simulink model "test_turb_sub"  (R2016a)
settings: Solver=VariableStepAuto  StartTime=0.0  StopTime=20  MaxStep=1e-3  RelTol=1e-3
libraries: simCryogenics_lib x12, nesl_utility x12, simulink x1
settings Model: Creator=FB229602  LastModifiedBy=FB229602
settings SimscapeCC: SimscapeLogType=all  SimscapeLogLimitData=off

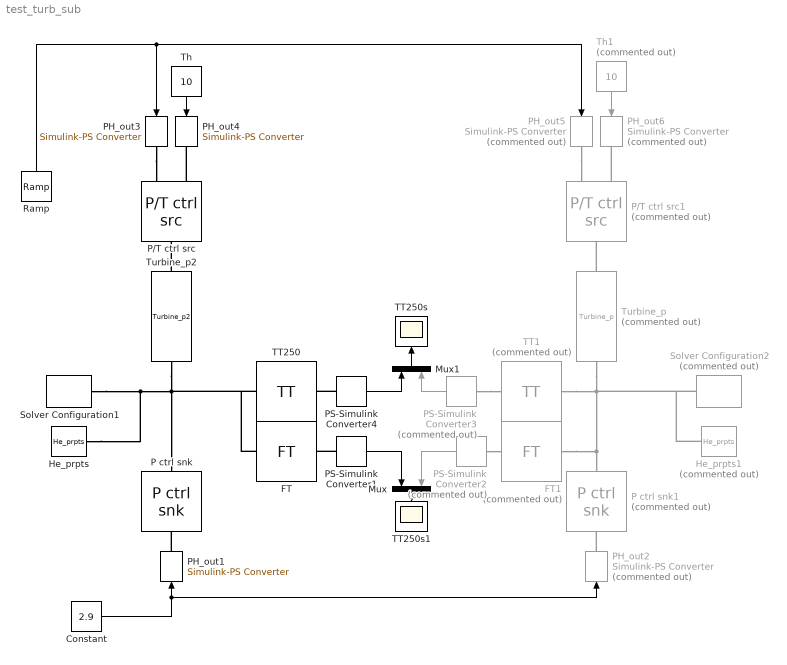
== system test_turb_sub ==
  Constant : Constant  Value=2.9
  FT : simCryogenics_lib/Sensors/FT
  FT1 : simCryogenics_lib/Sensors/FT  Commented=on
  He_prpts : simCryogenics_lib/Utilities/He_prpts  P_min=0.25 bar  P_max=20 bar  T_min=3 K  T_max=320 K  N=100  Mol=4.0026 * 10 ^ (- 3) kg/mol
  He_prpts1 : simCryogenics_lib/Utilities/He_prpts  Commented=on  P_min=0.25 bar  P_max=20 bar  T_min=3 K  T_max=320 K  N=100  Mol=4.0026 * 10 ^ (- 3) kg/mol
  Mux : Mux  Inputs=2
  Mux1 : Mux  Inputs=2
  P ctrl snk : simCryogenics_lib/Sources_Sinks/P ctrl snk
  P ctrl snk1 : simCryogenics_lib/Sources_Sinks/P ctrl snk  Commented=on
  P/T ctrl src : simCryogenics_lib/Sources_Sinks/P//T ctrl src
  P/T ctrl src1 : simCryogenics_lib/Sources_Sinks/P//T ctrl src  Commented=on
  PH_out1 : nesl_utility/Simulink-PS Converter  PhysicalDomain=network_engine_domain  SubClassName=ps_input  LeftPortType=input  RightPortType=output  PseudoPeriodic=off  Frequencies=[]  NoiseDistribution=none  NoiseParameters=[]  Unit=1  AffineConversion=off  InputFiltering=off  SimscapeFilterOrder=1  InputFilterTimeConstant=0.001  UdotUserProvided=1
  PH_out2 : nesl_utility/Simulink-PS Converter  Commented=on  PhysicalDomain=network_engine_domain  SubClassName=ps_input  LeftPortType=input  RightPortType=output  PseudoPeriodic=off  Frequencies=[]  NoiseDistribution=none  NoiseParameters=[]  Unit=1  AffineConversion=off  InputFiltering=off  SimscapeFilterOrder=1  InputFilterTimeConstant=0.001  UdotUserProvided=1
  PH_out3 : nesl_utility/Simulink-PS Converter  PhysicalDomain=network_engine_domain  SubClassName=ps_input  LeftPortType=input  RightPortType=output  PseudoPeriodic=off  Frequencies=[]  NoiseDistribution=none  NoiseParameters=[]  Unit=bar  AffineConversion=off  InputFiltering=off  SimscapeFilterOrder=1  InputFilterTimeConstant=0.001  UdotUserProvided=1
  PH_out4 : nesl_utility/Simulink-PS Converter  PhysicalDomain=network_engine_domain  SubClassName=ps_input  LeftPortType=input  RightPortType=output  PseudoPeriodic=off  Frequencies=[]  NoiseDistribution=none  NoiseParameters=[]  Unit=K  AffineConversion=off  InputFiltering=off  SimscapeFilterOrder=1  InputFilterTimeConstant=0.001  UdotUserProvided=1
  PH_out5 : nesl_utility/Simulink-PS Converter  Commented=on  PhysicalDomain=network_engine_domain  SubClassName=ps_input  LeftPortType=input  RightPortType=output  PseudoPeriodic=off  Frequencies=[]  NoiseDistribution=none  NoiseParameters=[]  Unit=bar  AffineConversion=off  InputFiltering=off  SimscapeFilterOrder=1  InputFilterTimeConstant=0.001  UdotUserProvided=1
  PH_out6 : nesl_utility/Simulink-PS Converter  Commented=on  PhysicalDomain=network_engine_domain  SubClassName=ps_input  LeftPortType=input  RightPortType=output  PseudoPeriodic=off  Frequencies=[]  NoiseDistribution=none  NoiseParameters=[]  Unit=K  AffineConversion=off  InputFiltering=off  SimscapeFilterOrder=1  InputFilterTimeConstant=0.001  UdotUserProvided=1
  PS-Simulink Converter1 : nesl_utility/PS-Simulink Converter  PhysicalDomain=network_engine_domain  SubClassName=ps_output  LeftPortType=input  RightPortType=output  PseudoPeriodic=off  Frequencies=[]  Unit=1  AffineConversion=off
  PS-Simulink Converter2 : nesl_utility/PS-Simulink Converter  Commented=on  PhysicalDomain=network_engine_domain  SubClassName=ps_output  LeftPortType=input  RightPortType=output  PseudoPeriodic=off  Frequencies=[]  Unit=1  AffineConversion=off
  PS-Simulink Converter3 : nesl_utility/PS-Simulink Converter  Commented=on  PhysicalDomain=network_engine_domain  SubClassName=ps_output  LeftPortType=input  RightPortType=output  PseudoPeriodic=off  Frequencies=[]  Unit=1  AffineConversion=off
  PS-Simulink Converter4 : nesl_utility/PS-Simulink Converter  PhysicalDomain=network_engine_domain  SubClassName=ps_output  LeftPortType=input  RightPortType=output  PseudoPeriodic=off  Frequencies=[]  Unit=1  AffineConversion=off
  Ramp : simulink/Sources/Ramp  slope=-1  start=0  X0=18
  Solver Configuration1 : nesl_utility/Solver Configuration  PhysicalDomain=network_engine_domain  SubClassName=solver  LeftPortType=input  RightPortType=generic  Accelerate=off  Tones=[]  Harmonics=[]  SimulateNoise=off  Profile=off  UseLocalSampling=off  EnableSwitchedLinearOptims=on  FrequencyDomain=off  UseCCode=off  RelTol=0.001  AbsTol=1e-06  MinStep=1e-09  ToWorkspace=off  RevertToSquareIcSolve=off  NumHomotopyIterations=100  PhasorMode=off  PhasorModeNumHarmonics=1  OverrideAbsTol=off  DoDC=off  ResidualTolerance=1e-09  UseLocalSolver=off  LocalSolverChoice=NE_BACKWARD_EULER_ADVANCER  LocalSolverSampleTime=20  DoFixedCost=off  MaxNonlinIter=10  MaxModeIter=2  LinearAlgebra=Sparse  DelaysMemoryBudget=1024  AutomaticFiltering=on  FilteringTimeConstant=0.001
  Solver Configuration2 : nesl_utility/Solver Configuration  Commented=on  PhysicalDomain=network_engine_domain  SubClassName=solver  LeftPortType=input  RightPortType=generic  Accelerate=off  Tones=[]  Harmonics=[]  SimulateNoise=off  Profile=off  UseLocalSampling=off  EnableSwitchedLinearOptims=on  FrequencyDomain=off  UseCCode=off  RelTol=0.001  AbsTol=1e-06  MinStep=1e-09  ToWorkspace=off  RevertToSquareIcSolve=off  NumHomotopyIterations=100  PhasorMode=off  PhasorModeNumHarmonics=1  OverrideAbsTol=off  DoDC=off  ResidualTolerance=1e-09  UseLocalSolver=off  LocalSolverChoice=NE_BACKWARD_EULER_ADVANCER  LocalSolverSampleTime=20  DoFixedCost=off  MaxNonlinIter=10  MaxModeIter=2  LinearAlgebra=Sparse  DelaysMemoryBudget=1024  AutomaticFiltering=on  FilteringTimeConstant=0.001
  TT1 : simCryogenics_lib/Sensors/TT  Commented=on
  TT250 : simCryogenics_lib/Sensors/TT
  TT250s : Scope
  TT250s1 : Scope
  Th : Constant  Value=10
  Th1 : Constant  Commented=on  Value=10
  Turbine_p : simCryogenics_lib/Elements/Turbine_p  Commented=on  A=5e-6 m^2  D=0.0255 m  Mass=0.02 kg  cst_eff=0  eta0=0.8  Tin0=20 K  Pin0=16 bar  Pout0=1.2 bar  N0=2250 1/s  Q0=0 W  v0=0  I=0 kg*m^2  gamma_specify=off  gamma_priority=None  gamma=0  C_specify=off  C_priority=None  C=0  Z_specify=off  Z_priority=None  Z=0  Cp_specify=off  Cp_priority=None  Cp=0 kJ/kg/K  Sin_specify=off  Sin_priority=None  Sin=0 kJ/kg  T_specify=off  T_priority=None  T=0 K  HoutIs_specify=off  HoutIs_priority=None  HoutIs=0 kJ/kg  u1_specify=off  u1_priority=None  u1=0 m/s  c1_specify=off  c1_priority=None  c1=0 m/s  v_specify=off  v_priority=None  v=0  eta_specify=off  eta_priority=None  eta=0  eta_var_specify=off  eta_var_priority=None  eta_var=0  N_specify=off  N_priority=None  N=0 rad/s  Q_specify=off  Q_priority=None  Q=0 W
  Turbine_p2 : simCryogenics_lib/Elements/Turbine_p2  A=5e-6 m^2  D=0.0255 m  Mass=0.02 kg  cst_eff=0  eta0=0.8  Tin0=20 K  Pin0=16 bar  Pout0=1.2 bar  N0=2250 1/s  Q0=0 W  v0=0  I=0 kg*m^2  gamma_specify=off  gamma_priority=None  gamma=0  C_specify=off  C_priority=None  C=0  Z_specify=off  Z_priority=None  Z=0  Cp_specify=off  Cp_priority=None  Cp=0 kJ/kg/K  Sin_specify=off  Sin_priority=None  Sin=0 kJ/kg  T_specify=off  T_priority=None  T=0 K  HoutIs_specify=off  HoutIs_priority=None  HoutIs=0 kJ/kg  u1_specify=off  u1_priority=None  u1=0 m/s  c1_specify=off  c1_priority=None  c1=0 m/s  v_specify=off  v_priority=None  v=0  eta_specify=off  eta_priority=None  eta=0  eta_var_specify=off  eta_var_priority=None  eta_var=0  N_specify=off  N_priority=None  N=0 rad/s  Q_specify=off  Q_priority=None  Q=0 W  rp_crit_specify=off  rp_crit_priority=None  rp_crit=1  rp_c_specify=off  rp_c_priority=None  rp_c=1
  wires:
  PS-Simulink Converter4/1 -> Mux1/1
  Th/1 -> PH_out4/1
  Ramp/1 -> PH_out5/1, PH_out3/1
  PS-Simulink Converter1/1 -> Mux/1
  Th1/1 -> PH_out6/1
  Constant/1 -> PH_out2/1, PH_out1/1
  Mux/1 -> TT250s1/1
  PS-Simulink Converter2/1 -> Mux/2
  Mux1/1 -> TT250s/1
  PS-Simulink Converter3/1 -> Mux1/2
  connections:
  Turbine_p2/LConn1 -- P/T ctrl src/RConn1
  PS-Simulink Converter4/LConn1 -- TT250/RConn1
  PH_out3/RConn1 -- P/T ctrl src/LConn1
  P/T ctrl src/LConn2 -- PH_out4/RConn1
  Solver Configuration1/RConn1 -- He_prpts/RConn1 -- Turbine_p2/RConn1 -- FT/LConn1 -- TT250/LConn1 -- P ctrl snk/RConn1
  PH_out1/RConn1 -- P ctrl snk/LConn1
  PS-Simulink Converter1/LConn1 -- FT/RConn1
  PS-Simulink Converter2/LConn1 -- FT1/RConn1
  Turbine_p/LConn1 -- P/T ctrl src1/RConn1
  PS-Simulink Converter3/LConn1 -- TT1/RConn1
  PH_out5/RConn1 -- P/T ctrl src1/LConn1
  P/T ctrl src1/LConn2 -- PH_out6/RConn1
  PH_out2/RConn1 -- P ctrl snk1/LConn1
  Turbine_p/RConn1 -- TT1/LConn1 -- He_prpts1/RConn1 -- Solver Configuration2/RConn1 -- FT1/LConn1 -- P ctrl snk1/RConn1
